simulink model "sdtwin_battery_full_cycles"  (R2026b)
settings: Solver=ode45  StartTime=0  StopTime=36000  MaxStep=1  RelTol=1e-9  AbsTol=1e-11
PostLoadFcn:
  | load(fullfile(fileparts(get_param(bdroot,'FileName')),'full_cycle_initial_config.mat'));
values from neighbouring files (symbols this model uses):
  command_current = 0.276484749523    [full_cycle_initial_config.mat]    (also in run_full_cycles_simulink.m = c.current_magnitude_A)
  initial_energy = [0 0]    [full_cycle_initial_config.mat]    (also in run_full_cycles_simulink.m = [0;0])
  initial_state = [0.9 0.27]    [full_cycle_initial_config.mat]    (also in run_full_cycles_simulink.m = [c.initial_xn;c.initial_xp])
settings Model: Creator=markl  LastModifiedBy=markl
settings DataIOCC: OutputOption=SpecifiedOutputTimes  OutputTimes=0:1:36000  SaveOutput=off

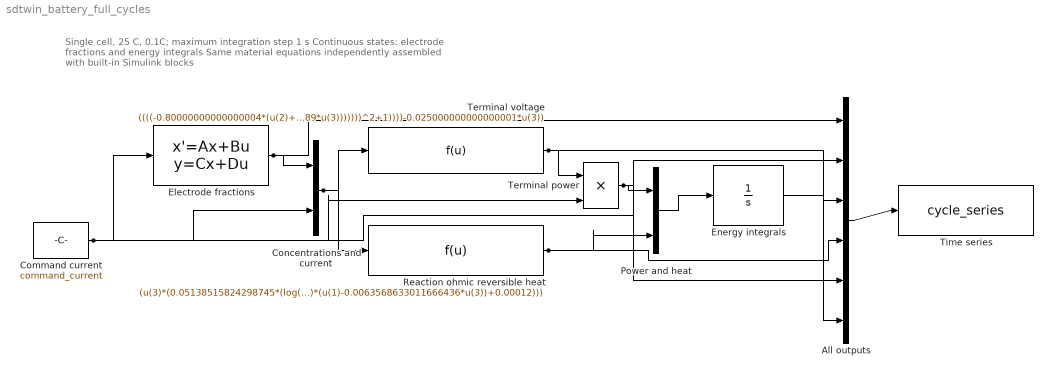
== system sdtwin_battery_full_cycles ==
  note: Single cell, 25 C, 0.1C; maximum integration step 1 s
      | Continuous states: electrode fractions and energy integrals
      | Same material equations independently assembled with built-in Simulink blocks
  All outputs : Mux  Inputs=6
  Command current : Constant  Value=command_current
  Concentrations and current : Mux  Inputs=2
  Electrode fractions : StateSpace  A=zeros(2)  B=[-8.7406870391041355e-05;5.4974842697313283e-05]  C=eye(2)  D=zeros(2,1)  InitialCondition=initial_state
  Energy integrals : Integrator  InitialCondition=initial_energy
  Power and heat : Mux  Inputs=2
  Reaction ohmic reversible heat : Fcn  Expr=(u(3)*(0.05138515824298745*(log((u(3)/(2*(5*sqrt((u(1)-0.0063568633011666436*u(3))*(1-(u(1)-0.0063568633011666436*u(3)))))))+sqrt((u(3)/(2*(5*sqrt((u(1)-0.0063568633011666436*u(3))*(1-(u(1)-0.0063568633011666436*u(3)))))))^2+1))+log((u(3)/(2*(6*sqrt((u(2)+0.0091624737828855489*u(3))*(1-(u(2)+0.0091624737828855489*u(3)))))))+sqrt((u(3)/(2*(6*sqrt((u(2)+0.0091624737828855489*u(3))*(1-(u(2)+0.0091624737828855489*u(3)))))))^2+1))))+0.025000000000000001*u(3)^2-u(3)*298.14999999999998*((((0*(u(2)+0.0091624737828855489*u(3))+0)*(u(2)+0.0091624737828855489*u(3))+4.0000000000000003e-05)*(u(2)+0.0091624737828855489*u(3))+-6.0000000000000002e-05)-(((0*(u(1)-0.0063568633011666436*u(3))+0.00014999999999999999)*(u(1)-0.0063568633011666436*u(3))+-0.00029999999999999997)*(u(1)-0.0063568633011666436*u(3))+0.00012)))
  Terminal power : Product  Inputs=**
  Terminal voltage : Fcn  Expr=((((-0.80000000000000004*(u(2)+0.0091624737828855489*u(3))+0.90000000000000002)*(u(2)+0.0091624737828855489*u(3))+-1.3)*(u(2)+0.0091624737828855489*u(3))+4.5999999999999996)-(((-0.94999999999999996*(u(1)-0.0063568633011666436*u(3))+2)*(u(1)-0.0063568633011666436*u(3))+-1.6000000000000001)*(u(1)-0.0063568633011666436*u(3))+0.65000000000000002)-(0.05138515824298745*(log((u(3)/(2*(5*sqrt((u(1)-0.0063568633011666436*u(3))*(1-(u(1)-0.0063568633011666436*u(3)))))))+sqrt((u(3)/(2*(5*sqrt((u(1)-0.0063568633011666436*u(3))*(1-(u(1)-0.0063568633011666436*u(3)))))))^2+1))+log((u(3)/(2*(6*sqrt((u(2)+0.0091624737828855489*u(3))*(1-(u(2)+0.0091624737828855489*u(3)))))))+sqrt((u(3)/(2*(6*sqrt((u(2)+0.0091624737828855489*u(3))*(1-(u(2)+0.0091624737828855489*u(3)))))))^2+1))))-0.025000000000000001*u(3))
  Time series : ToWorkspace  VariableName=cycle_series  SaveFormat=Structure With Time  SampleTime=-1
  wires:
  Command current/1 -> Electrode fractions/1, Concentrations and current/2, Terminal power/2, All outputs/2
  Electrode fractions/1 -> Concentrations and current/1, All outputs/1
  Concentrations and current/1 -> Terminal voltage/1, Reaction ohmic reversible heat/1
  Terminal voltage/1 -> Terminal power/1, All outputs/3
  Terminal power/1 -> Power and heat/1, All outputs/5
  Reaction ohmic reversible heat/1 -> Power and heat/2, All outputs/4
  Power and heat/1 -> Energy integrals/1
  Energy integrals/1 -> All outputs/6
  All outputs/1 -> Time series/1
